simulink model "hack3"  (R2015a)
settings: Solver=ode45  StartTime=0.0  StopTime=7  RelTol=1e-3
values from neighbouring files (symbols this model uses):
  g = 9.81    [continuous_func_V2.m]    (also in parameters.mat)
  Ix = 0.005    [parameters.mat]
  Iy = 0.005    [parameters.mat]
  Iz = 0.009    [parameters.mat]
  m = 0.5    [parameters.mat]
settings Model: Creator=Craig  LastModifiedBy=Shazara Bassarath

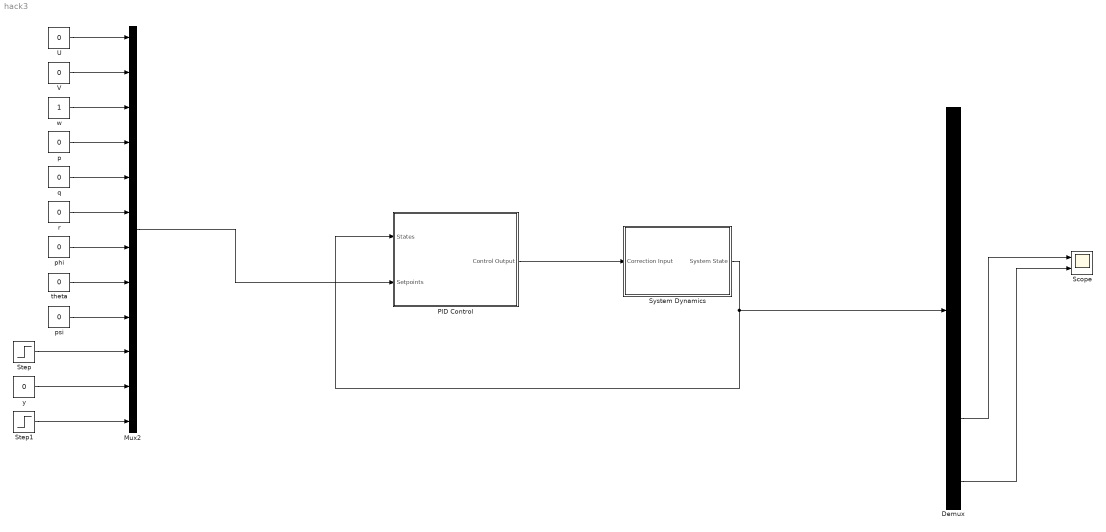
== system hack3 ==
  Demux : Demux  Outputs=12
  Mux2 : Mux  Inputs=12
  PID Control : Subsystem
  Scope : Scope  NumInputPorts=2
      settings: YMin=-0.775~100.425  YMax=-0.275~100.925
  Step : Step  Time=6  After=10  SampleTime=0
  Step1 : Step  After=100  SampleTime=0
  System Dynamics : Subsystem
  U : Constant  Value=0
  V : Constant  Value=0
  p : Constant  Value=0
  phi : Constant  Value=0
  psi : Constant  Value=0
  q : Constant  Value=0
  r : Constant  Value=0
  theta : Constant  Value=0
  w : Constant
  y : Constant  Value=0
  wires:
  PID Control/1(Control Output) -> System Dynamics/1(Correction Input)
  System Dynamics/1(System State) -> PID Control/1(States), Demux/1
  U/1 -> Mux2/1
  V/1 -> Mux2/2
  w/1 -> Mux2/3
  p/1 -> Mux2/4
  q/1 -> Mux2/5
  r/1 -> Mux2/6
  phi/1 -> Mux2/7
  psi/1 -> Mux2/9
  theta/1 -> Mux2/8
  Mux2/1 -> PID Control/2(Setpoints)
  Step/1 -> Mux2/10
  y/1 -> Mux2/11
  Step1/1 -> Mux2/12
  Demux/12 -> Scope/2
  Demux/10 -> Scope/1

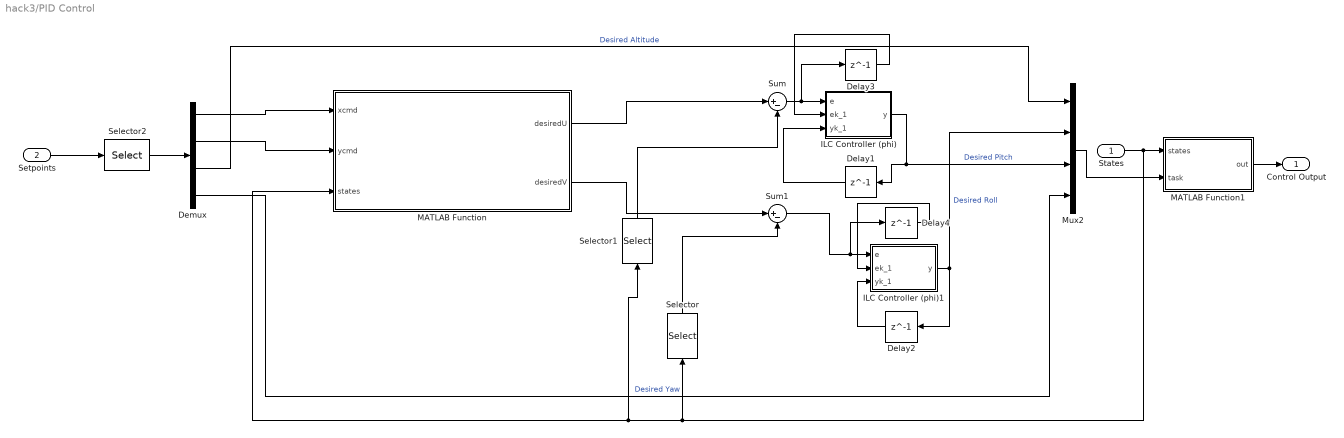
== system hack3/PID Control ==
  States : Inport
  Setpoints : Inport  Port=2
  Delay{1..4} (4 alike) : Delay  DelayLength=1  SampleTime=1e-4
  Demux : Demux
  ILC Controller (phi) : MATLAB Function  TreatAsAtomicUnit=on  SystemSampleTime=1e-4
  ILC Controller (phi)1 : MATLAB Function  TreatAsAtomicUnit=on  SystemSampleTime=1e-4
  MATLAB Function : MATLAB Function  TreatAsAtomicUnit=on
  MATLAB Function1 : MATLAB Function  TreatAsAtomicUnit=on
  Mux2 : Mux
  Selector : Selector  InputPortWidth=12  Indices=[2]
  Selector1 : Selector  InputPortWidth=12  Indices=[1]
  Selector2 : Selector  InputPortWidth=12  Indices=[10 11 12 9]
  Sum : Sum  Inputs=|+-
  Sum1 : Sum  Inputs=|+-
  Control Output : Outport
  wires:
  Selector/1 -> Sum1/2
  ILC Controller (phi)1/1(y) -> Delay2/1, Mux2/2  "Desired Roll"
  MATLAB Function/2(desiredV) -> Sum1/1
  Selector1/1 -> Sum/2
  Mux2/1 -> MATLAB Function1/2(task)
  MATLAB Function/1(desiredU) -> Sum/1
  Demux/3 -> Mux2/1  "Desired Altitude"
  Selector2/1 -> Demux/1
  MATLAB Function1/1(out) -> Control Output/1
  Demux/4 -> Mux2/4  "Desired Yaw"
  States/1 -> Selector/1, Selector1/1, MATLAB Function/3(states), MATLAB Function1/1(states)
  Demux/1 -> MATLAB Function/1(xcmd)
  Demux/2 -> MATLAB Function/2(ycmd)
  ILC Controller (phi)/1(y) -> Delay1/1, Mux2/3  "Desired Pitch"
  Setpoints/1 -> Selector2/1
  Sum/1 -> Delay3/1, ILC Controller (phi)/1(e)
  Delay1/1 -> ILC Controller (phi)/3(yk_1)
  Delay2/1 -> ILC Controller (phi)1/3(yk_1)
  Sum1/1 -> Delay4/1, ILC Controller (phi)1/1(e)
  Delay3/1 -> ILC Controller (phi)/2(ek_1)
  Delay4/1 -> ILC Controller (phi)1/2(ek_1)

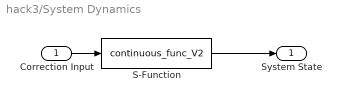
== system hack3/System Dynamics ==
  Correction Input : Inport
  S-Function : S-Function  FunctionName=continuous_func_V2  Parameters=m,Ix,Iy,Iz
  System State : Outport
  wires:
  S-Function/1 -> System State/1
  Correction Input/1 -> S-Function/1

== matlab function hack3/PID Control/MATLAB Function1 ==
  data m settings: description=Mass of the quadrotor.
  data g settings: description=Gavitational acceleration
  data Ix settings: description=Inertia matrix x component.
  data Iy settings: description=Inertia matrix y component.
  data Iz settings: description=Inertia matrix z component.
  data: states input; task input; out output; m parameter; g parameter; Ix parameter; Iy parameter; Iz parameter
function out=control(states, task, m, g, Ix, Iy, Iz)
% ----------------------------------------------------
% This script applies the control laws to the input
% data inferred from the sensors to obtain the values
% of the four control variables Ui.
% ----------------------------------------------------
%#codegen

%Linear Velocity Components
%u=states(1); %This is effectively U
%v=states(2); %V
w=states(3); %W

%Angular Velocity Components
p=states(4); %P
q=states(5); %Q
r=states(6); %R

%Euler Angles
phi=states(7);
theta=states(8);
psi=states(9);

%Linear Positions
%x=states(10);
%y=states(11);
z=states(12);

% Task data
heightd = task(1);
rolld = task(2);
pitchd = task(3);
yawd = task(4);

% Control parameters
k1 = 4;
k2 = 2;
k3 = 4;
k4 = 2;
k5 = 2;
k6 = 2;
k7 = 2;
k8 = 2;

% Control laws
control_1 = -k1*(z - heightd) - k2*w;
U1 = (m*g+control_1)/(cos(phi)*cos(theta)); 
U2 = Ix*(-k3*(phi - rolld) - k4*p);
U3 = Iy*(-k5*(theta - pitchd) - k6*q);
U4 = Iz*(-k7*(psi - yawd) - k8*r);

out = zeros(4,1);
out(1) = U1;
out(2) = U2;
out(3) = U3;
out(4) = U4;

== matlab function hack3/PID Control/MATLAB Function ==
  data: xcmd input; desiredU output; ycmd input; states input; desiredV output
function [desiredU,desiredV] = translation(xcmd,ycmd,states)
%This function is used to determine the desired velocities that can enable
%the position control of the quadcopter
psi=states(9);
x=states(10);
y=states(11);

Xerr=xcmd-x;
Yerr=ycmd-y;

desiredU=Xerr*cos(psi)+Yerr*sin(psi); %Desired U is the desired velocity in the X direction of the body frame

desiredV=Yerr*cos(psi)-Xerr*sin(psi);%This is the desired velocity in the Y direction of the body frame

== matlab function hack3/PID Control/ILC Controller (phi) ==
  data: e input; ek_1 input; y output; yk_1 input
function y = fcn(e , ek_1, yk_1)
%#codegen

for i=1:1

y = yk_1 + 0.5*(e - 0.001*ek_1) ; end

== matlab function hack3/PID Control/ILC Controller (phi)1 ==
  data: e input; ek_1 input; y output; yk_1 input
function y = fcn(e , ek_1, yk_1)
%#codegen

for i=1:1

y = yk_1 + 0.5*(e - 0.001*ek_1); end
